simulink model "Sensor_estimator_model_simulink_1_3"  (R2025b)
settings: Solver=VariableStepAuto  StartTime=0.0  StopTime=10.0  RelTol=1e-3
undefined symbols (not defined in the file or in its folder): sigma_m_square, taue, taum
settings Model: Creator=flori  LastModifiedBy=flori

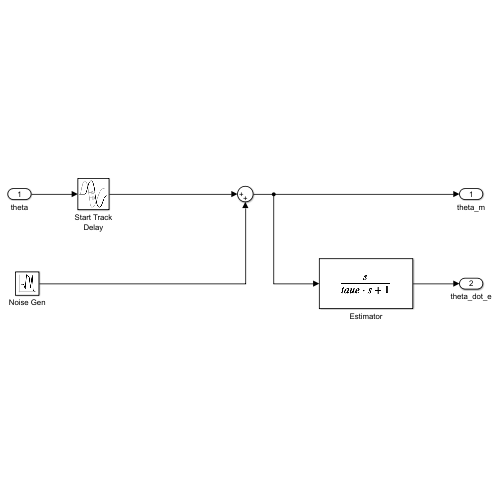
[thumbnail: Simulink's stored preview of the top-level diagram]
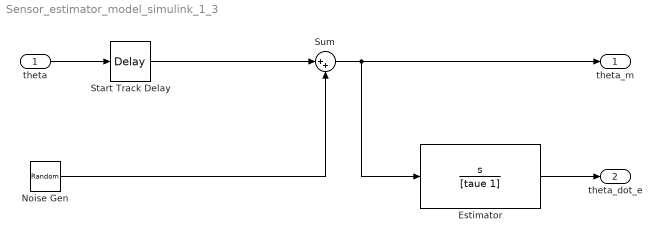
== system Sensor_estimator_model_simulink_1_3 ==
  theta : Inport
  Estimator : TransferFcn  Numerator=[1 0]  Denominator=[taue 1]
  Noise Gen : RandomNumber  Variance=sigma_m_square  SampleTime=0.01
  Start Track Delay : TransportDelay  DelayTime=taum
  Sum : Sum  Inputs=|++
  theta_m : Outport
  theta_dot_e : Outport  Port=2
  wires:
  theta/1 -> Start Track Delay/1
  Start Track Delay/1 -> Sum/1
  Estimator/1 -> theta_dot_e/1
  Sum/1 -> theta_m/1, Estimator/1
  Noise Gen/1 -> Sum/2
